simulink library "soar_interface_lib"  (R2018b)
settings: Solver=VariableStepAuto  StartTime=0.0  StopTime=10.0  RelTol=1e-3
undefined symbols (not defined in the file): soarParams
libraries: simulink x2, dspswit3 x1, soar_interp x1, soar_lib x1
settings Model: Creator=taylorreynolds  LastModifiedBy=Taylor
settings SFSimCC: SimUseLocalCustomCode=off
settings RTWCC: RTWUseLocalCustomCode=off
settings CodeAppCC: StateflowObjectComments=on

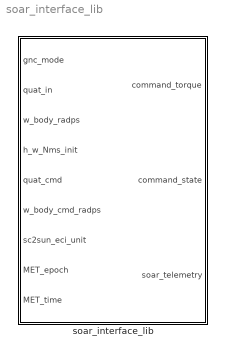
== system soar_interface_lib ==
  soar_interface_lib : Subsystem

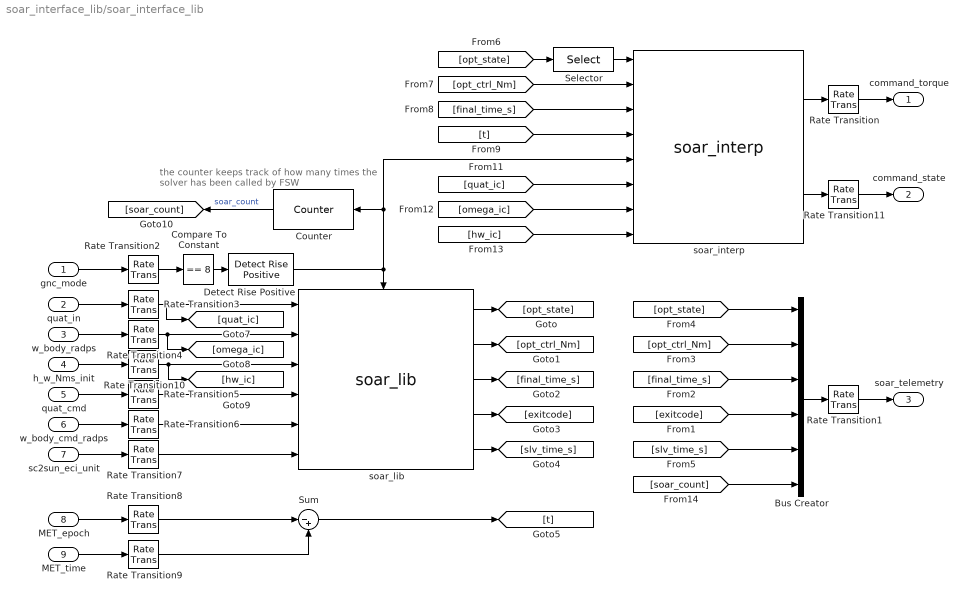
== system soar_interface_lib/soar_interface_lib ==
  note: the counter keeps track of how many times
      | the solver has been called by FSW
  gnc_mode : Inport
  quat_in : Inport  Port=2
  w_body_radps : Inport  Port=3
  h_w_Nms_init : Inport  Port=4
  quat_cmd : Inport  Port=5
  w_body_cmd_radps : Inport  Port=6
  sc2sun_eci_unit : Inport  Port=7
  MET_epoch : Inport  Port=8
  MET_time : Inport  Port=9
  Bus Creator : BusCreator  Inputs=6  OutDataTypeStr=Bus: soar_telemetry
      settings: InheritFromInputs=off
  Compare To Constant : simulink/Logic and Bit Operations/Compare To Constant  relop===  const=8  OutDataTypeStr=boolean
  Counter : dspswit3/Counter  Direction=Up  CountEvent=Rising edge  CounterSize=32 bits  MaxCount=255  InitialCount=0  Output=Count  HitValue=32  ResetInput=off  SamplesPerFrame=1  Ts=1  CntDtype=uint32  HitDtype=Logical
  Detect Rise Positive : simulink/Logic and Bit Operations/Detect Rise Positive  vinit=0  OutDataTypeStr=boolean
  Rate Transition : RateTransition
  Rate Transition1 : RateTransition  OutPortSampleTime=fswParams.sample_time_s
  Rate Transition{2,4,6..10} (7 alike) : RateTransition  OutPortSampleTime=soarParams.sample_time_s
  Rate Transition11 : RateTransition  InitialCondition=soarParams.ic.cmd_state
  Rate Transition3 : RateTransition  InitialCondition=soarParams.ic.quat_in  OutPortSampleTime=soarParams.sample_time_s
  Rate Transition5 : RateTransition  InitialCondition=soarParams.ic.quat_cmd  OutPortSampleTime=soarParams.sample_time_s
  Selector : Selector  InputPortWidth=10*soarParams.N  IndexOptions=Index vector (dialog)  Indices=[91 92 93 94 95 96 97 98 99 100]  OutputSizes=1
  Sum : Sum  Inputs=|-+
  soar_interp : soar_interp/soar_interp  SystemSampleTime=-1
  soar_lib : soar_lib/soar_lib  SystemSampleTime=-1
  command_torque : Outport
  command_state : Outport  Port=2
  soar_telemetry : Outport  Port=3  OutDataTypeStr=Bus: soar_telemetry
  wires:
  [soar_count] -> Bus Creator/6
  Rate Transition11/1 -> command_state/1
  Rate Transition/1 -> command_torque/1
  [hw_ic] -> soar_interp/8
  [omega_ic] -> soar_interp/7
  [quat_ic] -> soar_interp/6
  Detect Rise Positive/1 -> soar_lib/Trigger, soar_interp/5, Counter/1
  [t] -> soar_interp/4
  [final_time_s] -> soar_interp/3
  [opt_ctrl_Nm] -> soar_interp/2
  [opt_state] -> Selector/1
  Counter/1 -> [soar_count]  "soar_count"
  soar_interp/2 -> Rate Transition11/1
  soar_interp/1 -> Rate Transition/1
  Rate Transition2/1 -> Compare To Constant/1
  quat_in/1 -> Rate Transition3/1
  w_body_radps/1 -> Rate Transition4/1
  quat_cmd/1 -> Rate Transition5/1
  w_body_cmd_radps/1 -> Rate Transition6/1
  sc2sun_eci_unit/1 -> Rate Transition7/1
  gnc_mode/1 -> Rate Transition2/1
  Compare To Constant/1 -> Detect Rise Positive/1
  soar_lib/1 -> [opt_state]
  soar_lib/5 -> [slv_time_s]
  soar_lib/4 -> [exitcode]
  MET_epoch/1 -> Rate Transition8/1
  MET_time/1 -> Rate Transition9/1
  Sum/1 -> [t]
  Bus Creator/1 -> Rate Transition1/1
  [slv_time_s] -> Bus Creator/5
  [exitcode] -> Bus Creator/4
  [final_time_s] -> Bus Creator/3
  [opt_ctrl_Nm] -> Bus Creator/2
  [opt_state] -> Bus Creator/1
  Rate Transition1/1 -> soar_telemetry/1
  Rate Transition3/1 -> [quat_ic], soar_lib/1
  Rate Transition4/1 -> soar_lib/2, [omega_ic]
  Rate Transition5/1 -> soar_lib/4
  Rate Transition6/1 -> soar_lib/5
  Rate Transition7/1 -> soar_lib/6
  Rate Transition8/1 -> Sum/1
  Rate Transition9/1 -> Sum/2
  Rate Transition10/1 -> soar_lib/3, [hw_ic]
  h_w_Nms_init/1 -> Rate Transition10/1
  soar_lib/2 -> [opt_ctrl_Nm]
  soar_lib/3 -> [final_time_s]
  Selector/1 -> soar_interp/1
